simulink model "Function_Blocks"  (R2020b)
settings: Solver=FixedStepDiscrete  StartTime=0.0  StopTime=40  FixedStep=0.001  RelTol=1e-3
undefined symbols (not defined in the file): AA, C1, DiscIntNeverNeededParam, Error_Limit, kq, kqL
libraries: simulink x1, eeGeneralControl x1
(part 1 of 2)
settings Model: Creator=Jan Størbu  LastModifiedBy=Green Crane Testbed
settings DataIOCC: ReturnWorkspaceOutputs=off
settings DebuggingCC: BusObjectLabelMismatch=error  ArithmeticOperatorsInVariantConditions=warning
settings SFSimCC: SimUseLocalCustomCode=off  CustomCodeUndefinedFunction=UseInterfaceOnly
settings RTWCC: RTWUseLocalCustomCode=off
settings ConfigComp: PLC_TargetIDE=indraworks  PLC_ReuseMLFcnVariable=on  PLC_GenerateReport=off  PLC_LaunchReport=off

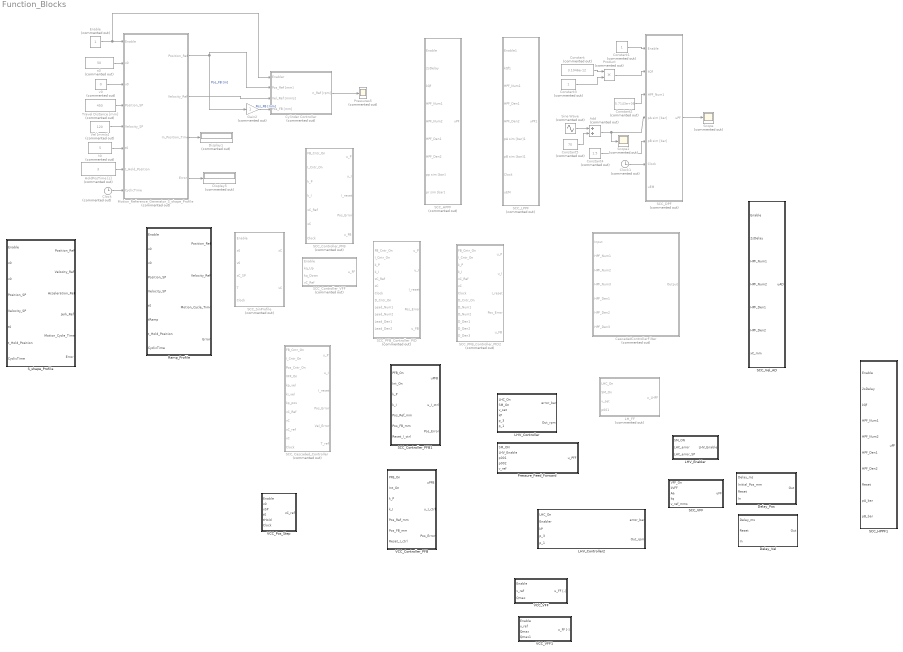
== system Function_Blocks ==
  Add : Sum  Commented=on
  CascadedControllerFilter : Subsystem  Commented=on  TreatAsAtomicUnit=on
  Clock : Clock  Commented=on
  Clock1 : Clock  Commented=on
  Constant : Constant  Commented=on  Value=3.1046e-12
  Constant1 : Constant  Commented=on  OutDataTypeStr=boolean
  Constant2 : Constant  Commented=on  Value=5.7143e+06
  Constant3 : Constant  Commented=on
  Constant4 : Constant  Commented=on  Value=1.5
  Constant5 : Constant  Commented=on  Value=70
  Cylinder Controller : Subsystem  Commented=on
  Delay_Pos : Subsystem  TreatAsAtomicUnit=on
  Delay_Vel : Subsystem  TreatAsAtomicUnit=on
  Display1 : Display  Commented=on
  Display5 : Display  Commented=on
  Enable : Constant  Commented=on  OutDataTypeStr=boolean
  Gain2 : Gain  Commented=on
  HoldPosTime [s] : Constant  Commented=on  Value=3
  "LHV_Controller " : Subsystem  TreatAsAtomicUnit=on
  LHV_Controller2 : Subsystem  TreatAsAtomicUnit=on
  LHV_Enabler : Subsystem  TreatAsAtomicUnit=on
  "LH_FF " : Subsystem  Commented=on
  Motion_Reference_Generator_S_shape_Profile : Subsystem  Commented=on  TreatAsAtomicUnit=on  VariantControl=S_shape_Profile
  Pressure_Feed_Forward : Subsystem  TreatAsAtomicUnit=on
  Pressures5 : Scope  Commented=on
  Product : Product  Commented=on
  Ramp_Profile : Subsystem  TreatAsAtomicUnit=on  VariantControl=Ramp_Profile
  SCC_Cascaded_Controller : Subsystem  Commented=on  TreatAsAtomicUnit=on
  SCC_Controller_PFB : Subsystem  Commented=on  TreatAsAtomicUnit=on
  SCC_Controller_PFB1 : Subsystem  TreatAsAtomicUnit=on
  SCC_Controller_VFF : Subsystem  Commented=on  TreatAsAtomicUnit=on
  SCC_DPF : Subsystem  Commented=on  TreatAsAtomicUnit=on
  SCC_HPPF : Subsystem  Commented=on  TreatAsAtomicUnit=on
  SCC_HPPF1 : Subsystem  TreatAsAtomicUnit=on
  SCC_LPPF : Subsystem  Commented=on  TreatAsAtomicUnit=on
  SCC_PFB_Controller_PID : Subsystem  Commented=on  TreatAsAtomicUnit=on
  SCC_PFB_Controller_PID2 : Subsystem  Commented=on  TreatAsAtomicUnit=on
  SCC_SinProfile : Subsystem  Commented=on  TreatAsAtomicUnit=on
  "SCC_VFF " : Subsystem  TreatAsAtomicUnit=on
  SCC_Vel_AD : Subsystem  TreatAsAtomicUnit=on
  S_shape_Profile : Subsystem  TreatAsAtomicUnit=on  VariantControl=S_shape_Profile
  Scope : Scope  Commented=on
  Scope1 : Scope  Commented=on
  Sine Wave : Sin  Commented=on  Amplitude=10  Frequency=14.5  SampleTime=0
  Travel Distance [mm] : Constant  Commented=on  Value=450
  VCC_Controller_PFB : Subsystem  TreatAsAtomicUnit=on
  VCC_Pos_Step : Subsystem  TreatAsAtomicUnit=on
  VCC_VFF : Subsystem  TreatAsAtomicUnit=on
  VCC_VFF1 : Subsystem  TreatAsAtomicUnit=on
  Vel [mm/s] : Constant  Commented=on  Value=120
  s0 : Constant  Commented=on  Value=50
  t0 : Constant  Commented=on  Value=5
  v0 : Constant  Commented=on  Value=0
  wires:
  Vel [mm/s]/1 -> Motion_Reference_Generator_S_shape_Profile/5(Velocity_SP)
  Gain2/1 -> Cylinder Controller/4(Pos_FB [mm])  "Pos_FB [mm]"
  Travel Distance [mm]/1 -> Motion_Reference_Generator_S_shape_Profile/4(Position_SP)
  Motion_Reference_Generator_S_shape_Profile/4(Error) -> Display5/1
  Enable/1 -> Motion_Reference_Generator_S_shape_Profile/1(Enable), Cylinder Controller/1(Enabler)
  Clock/1 -> Motion_Reference_Generator_S_shape_Profile/8(CyclicTime)
  Motion_Reference_Generator_S_shape_Profile/3(" In_Position_Time") -> Display1/1
  Motion_Reference_Generator_S_shape_Profile/2(Velocity_Ref) -> Cylinder Controller/3(Vel_Ref [mm/s])
  Motion_Reference_Generator_S_shape_Profile/1(Position_Ref) -> Cylinder Controller/2(Pos_Ref [mm]), Gain2/1  "Pos_FB [m]"
  s0/1 -> Motion_Reference_Generator_S_shape_Profile/2(x0)
  v0/1 -> Motion_Reference_Generator_S_shape_Profile/3(v0)
  HoldPosTime [s]/1 -> Motion_Reference_Generator_S_shape_Profile/7(t_Hold_Position)
  t0/1 -> Motion_Reference_Generator_S_shape_Profile/6(t0)
  Cylinder Controller/1(n_Ref [rpm]) -> Pressures5/1
  Constant/1 -> Product/1
  Sine Wave/1 -> Add/1
  SCC_DPF/1(uPF) -> Scope/1
  Constant4/1 -> SCC_DPF/5(pB sim [bar])
  Constant2/1 -> SCC_DPF/3(HPF_Num1)
  Add/1 -> Scope1/1, SCC_DPF/4(pA sim [bar])
  Constant5/1 -> Add/2
  Constant1/1 -> SCC_DPF/1(Enable)
  Clock1/1 -> SCC_DPF/6(Clock)
  Constant3/1 -> Product/2
  Product/1 -> SCC_DPF/2(kQf)

== system Function_Blocks/CascadedControllerFilter ==
  Input : Inport
  HPF_Num1 : Inport  Port=2
  HPF_Num2 : Inport  Port=3
  HPF_Num3 : Inport  Port=4
  HPF_Den1 : Inport  Port=5
  HPF_Den2 : Inport  Port=6
  HPF_Den3 : Inport  Port=7
  HP_Filter : DiscreteTransferFcn  NumeratorSource=Input port  Numerator=[3.786e-11 -3.786e-11]  DenominatorSource=Input port  Denominator=[1 -0.9954]  SampleTime=0.001  a0EqualsOne=on
      settings: InputPortMap=u0,p1,p3
  Vector Concatenate : Concatenate  NumInputs=3
  Vector Concatenate1 : Concatenate  NumInputs=3
  Output : Outport  VectorParamsAs1DForOutWhenUnconnected=off
  wires:
  HPF_Num1/1 -> Vector Concatenate/1
  Input/1 -> HP_Filter/1
  HPF_Num3/1 -> Vector Concatenate/3
  HPF_Den1/1 -> Vector Concatenate1/1
  HPF_Num2/1 -> Vector Concatenate/2
  HPF_Den3/1 -> Vector Concatenate1/3
  HPF_Den2/1 -> Vector Concatenate1/2
  Vector Concatenate1/1 -> HP_Filter/3
  Vector Concatenate/1 -> HP_Filter/2
  HP_Filter/1 -> Output/1

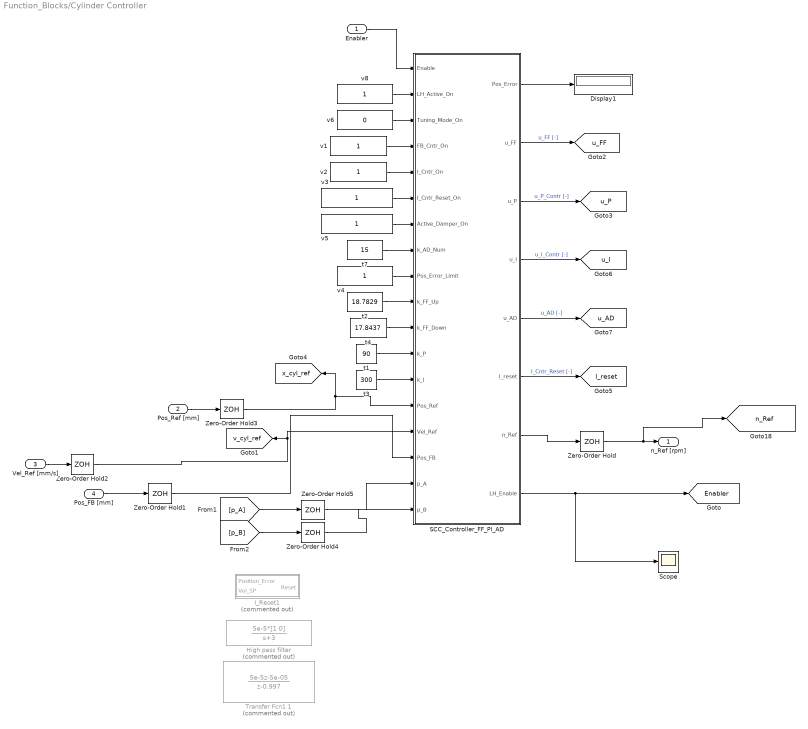
== system Function_Blocks/Cylinder Controller ==
  Enabler : Inport
  Pos_Ref [mm] : Inport  Port=2
  Vel_Ref [mm/s] : Inport  Port=3
  Pos_FB [mm] : Inport  Port=4
  Display1 : Display
  High pass filter : TransferFcn  Commented=on  Numerator=5e-5*[1 0]  Denominator=[1 3]
  I_Reset1 : Subsystem  Commented=on
  SCC_Controller_FF_PI_AD : Subsystem  TreatAsAtomicUnit=on
  Scope : Scope
  Transfer Fcn1 1 : DiscreteTransferFcn  Commented=on  Numerator=[5e-5 -5e-05]  Denominator=[1 -0.997]
  Zero-Order Hold{,1..5} (6 alike) : ZeroOrderHold  SampleTime=0.001
  t1 : Constant  Value=90
  t2 : Constant  Value=18.7829
  t3 : Constant  Value=300
  t4 : Constant  Value=17.8437
  t7 : Constant  Value=15
  v{1..3,5,8} (5 alike) : Constant  OutDataTypeStr=boolean
  v4 : Constant
  v6 : Constant  Value=0  OutDataTypeStr=boolean
  n_Ref [rpm] : Outport  VectorParamsAs1DForOutWhenUnconnected=off
  tag scope: Enabler=global, I_reset=global, n_Ref=global, u_AD=global, u_FF=global, u_I=global, u_P=global, v_cyl_ref=global, x_cyl_ref=global
  wires:
  v2/1 -> SCC_Controller_FF_PI_AD/5(I_Cntr_On)
  t3/1 -> SCC_Controller_FF_PI_AD/13(k_I)
  v1/1 -> SCC_Controller_FF_PI_AD/4(FB_Cntr_On)
  t1/1 -> SCC_Controller_FF_PI_AD/12(k_P)
  Pos_FB [mm]/1 -> Zero-Order Hold1/1
  SCC_Controller_FF_PI_AD/3(u_P) -> [u_P]  "u_P_Contr [-]"
  SCC_Controller_FF_PI_AD/2(u_FF) -> [u_FF]  "u_FF [-]"
  Pos_Ref [mm]/1 -> Zero-Order Hold3/1
  Vel_Ref [mm/s]/1 -> Zero-Order Hold2/1
  SCC_Controller_FF_PI_AD/6(I_reset) -> [I_reset]  "I_Cntr_Reset [-]"
  SCC_Controller_FF_PI_AD/1(Pos_Error) -> Display1/1
  SCC_Controller_FF_PI_AD/7(n_Ref) -> Zero-Order Hold/1
  SCC_Controller_FF_PI_AD/4(u_I) -> [u_I]  "u_I_Contr [-]"
  Zero-Order Hold/1 -> [n_Ref], n_Ref [rpm]/1
  Zero-Order Hold1/1 -> SCC_Controller_FF_PI_AD/16(Pos_FB)
  Zero-Order Hold2/1 -> SCC_Controller_FF_PI_AD/15(Vel_Ref), [v_cyl_ref]
  Zero-Order Hold3/1 -> SCC_Controller_FF_PI_AD/14(Pos_Ref), [x_cyl_ref]
  v3/1 -> SCC_Controller_FF_PI_AD/6(I_Cntr_Reset_On)
  v4/1 -> SCC_Controller_FF_PI_AD/9(Pos_Error_Limit)
  v5/1 -> SCC_Controller_FF_PI_AD/7(Active_Damper_On)
  [p_A] -> Zero-Order Hold5/1
  [p_B] -> Zero-Order Hold4/1
  Zero-Order Hold4/1 -> SCC_Controller_FF_PI_AD/18(p_B)
  Zero-Order Hold5/1 -> SCC_Controller_FF_PI_AD/17(p_A)
  SCC_Controller_FF_PI_AD/5(u_AD) -> [u_AD]  "u_AD [-]"
  t7/1 -> SCC_Controller_FF_PI_AD/8(k_AD_Num)
  v6/1 -> SCC_Controller_FF_PI_AD/3(Tuning_Mode_On)
  Enabler/1 -> SCC_Controller_FF_PI_AD/1(Enable)
  v8/1 -> SCC_Controller_FF_PI_AD/2(LH_Active_On)
  SCC_Controller_FF_PI_AD/8(LH_Enable) -> Scope/1, [Enabler]
  t2/1 -> SCC_Controller_FF_PI_AD/10(k_FF_Up)
  t4/1 -> SCC_Controller_FF_PI_AD/11(k_FF_Down)

== system Function_Blocks/Delay_Pos ==
  Delay_ms : Inport
  Initial_Pos_mm : Inport  Port=2
  Reset : Inport  Port=3  OutDataTypeStr=boolean
  In : Inport  Port=4
  Delay : Delay  DelayLengthSource=Input port  DelayLengthUpperLimit=200  InitialConditionSource=Input port  ExternalReset=Level hold  SampleTime=0.001
      settings: InputPortMap=u0,p1,r5,p4
  Out : Outport  VectorParamsAs1DForOutWhenUnconnected=off
  wires:
  Delay_ms/1 -> Delay/2
  Delay/1 -> Out/1
  In/1 -> Delay/1
  Reset/1 -> Delay/3
  Initial_Pos_mm/1 -> Delay/4

== system Function_Blocks/Delay_Vel ==
  Delay_ms : Inport
  Reset : Inport  Port=2  OutDataTypeStr=boolean
  In : Inport  Port=3
  Delay : Delay  DelayLengthSource=Input port  DelayLengthUpperLimit=200  ExternalReset=Level hold  SampleTime=0.001
      settings: InputPortMap=u0,p1,r5
  Out : Outport  VectorParamsAs1DForOutWhenUnconnected=off
  wires:
  Delay_ms/1 -> Delay/2
  Delay/1 -> Out/1
  In/1 -> Delay/1
  Reset/1 -> Delay/3

== system Function_Blocks/LHV_Controller  ==
  LHC_On : Inport  OutDataTypeStr=boolean
  SM_On : Inport  Port=2  OutDataTypeStr=boolean
  v_set : Inport  Port=3
  kP : Inport  Port=4
  p_3 : Inport  Port=5
  p_1 : Inport  Port=6
  1 : Gain  Gain=1e5
  12 : Gain  Gain=1e5
  Abs : Abs
  Add6 : Sum  Inputs=|+-
  Constant : Constant  Value=0
  Constant1 : Constant  Value=0
  Constant7 : Constant  Value=0
  Gain : Gain  Gain=1e-5
  Gain15 : Gain  Gain=60/(2*pi)
  Product : Product
  Saturation1 : Saturate  UpperLimit=1000  LowerLimit=-1000
  Switch1 : Switch  Criteria=u2 > Threshold
  Switch3 : Switch  Criteria=u2 > Threshold  OutDataTypeStr=boolean
  Switch5 : Switch  Criteria=u2 > Threshold
  Switch6 : Switch  Criteria=u2 > Threshold
  error_bar : Outport  VectorParamsAs1DForOutWhenUnconnected=off
  Out_rpm : Outport  Port=2  VectorParamsAs1DForOutWhenUnconnected=off
  wires:
  Product/1 -> Gain15/1  "Pa"
  Add6/1 -> Product/1, Gain/1  "FF+FB [rpm]"
  12/1 -> Add6/1
  Gain15/1 -> Switch1/1  "FF+FB [rpm]"
  p_3/1 -> Switch5/1  "[bar]"
  p_1/1 -> Switch6/1  "[bar]"
  1/1 -> Add6/2
  Constant/1 -> Switch1/3
  LHC_On/1 -> Switch1/2
  Switch1/1 -> Saturation1/1
  Saturation1/1 -> Out_rpm/1
  Constant7/1 -> Switch5/3, Switch6/3
  Switch3/1 -> Switch5/2, Switch6/2  "[bar]"
  Switch6/1 -> 1/1
  Switch5/1 -> 12/1
  Constant1/1 -> Switch3/1
  v_set/1 -> Abs/1
  Abs/1 -> Switch3/2
  SM_On/1 -> Switch3/3  "[bar]"
  Gain/1 -> error_bar/1
  kP/1 -> Product/2

== system Function_Blocks/LHV_Controller2 ==
  LHC_On : Inport  OutDataTypeStr=boolean
  Enabler : Inport  Port=2  OutDataTypeStr=boolean
  kP : Inport  Port=3
  p_3 : Inport  Port=4
  p_1 : Inport  Port=5
  1 : Gain  Gain=1e5
  12 : Gain  Gain=1e5
  Add1 : Sum  Inputs=|+-
  Add6 : Sum  Inputs=|+-
  Constant : Constant  Value=0
  Constant7 : Constant  Value=0
  Gain15 : Gain  Gain=60/(2*pi)
  Product : Product
  Saturation1 : Saturate  UpperLimit=1000  LowerLimit=0
  Switch1 : Switch  Criteria=u2 > Threshold
  Switch5 : Switch  Criteria=u2 > Threshold
  Switch6 : Switch  Criteria=u2 > Threshold
  "error_bar " : Outport  VectorParamsAs1DForOutWhenUnconnected=off
  Out_rpm : Outport  Port=2  VectorParamsAs1DForOutWhenUnconnected=off
  wires:
  Product/1 -> Gain15/1  "Pa"
  Add6/1 -> Product/1  "FF+FB [rpm]"
  12/1 -> Add6/1
  Gain15/1 -> Switch1/1  "FF+FB [rpm]"
  p_3/1 -> Add1/1, Switch5/1  "[bar]"
  p_1/1 -> Add1/2, Switch6/1  "[bar]"
  1/1 -> Add6/2
  Constant/1 -> Switch1/3
  LHC_On/1 -> Switch1/2
  Switch1/1 -> Saturation1/1
  Saturation1/1 -> Out_rpm/1
  Constant7/1 -> Switch5/3, Switch6/3
  Enabler/1 -> Switch5/2, Switch6/2  "[bar]"
  Switch6/1 -> 1/1
  Switch5/1 -> 12/1
  kP/1 -> Product/2
  Add1/1 -> "error_bar "/1  "FF+FB [rpm]"

== system Function_Blocks/LHV_Enabler ==
  SM_ON : Inport  OutDataTypeStr=boolean
  LHC_error : Inport  Port=2
  LHC_error_SP : Inport  Port=3
  MATLAB Function1 : MATLAB Function  TreatAsAtomicUnit=on
  LHV_Enable : Outport  VectorParamsAs1DForOutWhenUnconnected=off
  wires:
  MATLAB Function1/1(y) -> LHV_Enable/1
  SM_ON/1 -> MATLAB Function1/3(SM_ON)
  LHC_error/1 -> MATLAB Function1/1(LHC_error)
  LHC_error_SP/1 -> MATLAB Function1/2(LHC_error_SP)

== system Function_Blocks/LH_FF  ==
  LHC_On : Inport
  SM_On : Inport  Port=2
  v_set : Inport  Port=3
  p001 : Inport  Port=4
  12 : Gain  Gain=1e5
  Abs : Abs
  Constant : Constant  Value=0
  Constant7 : Constant  Value=0
  Switch1 : Switch  Criteria=u2 > Threshold
  Switch5 : Switch  Criteria=u2 > Threshold
  Transfer Fcn10 : TransferFcn  Numerator="[C1  kqL]"  Denominator=[0.002*kq kq ]
  u_LHFF : Outport  VectorParamsAs1DForOutWhenUnconnected=off
  wires:
  Transfer Fcn10/1 -> Switch1/1  "FF+FB [rpm]"
  p001/1 -> Switch5/1  "[bar]"
  Constant/1 -> Switch1/3
  LHC_On/1 -> Switch1/2
  Switch1/1 -> u_LHFF/1
  Constant7/1 -> Switch5/3
  Abs/1 -> Switch5/2  "[bar]"
  Switch5/1 -> 12/1
  12/1 -> Transfer Fcn10/1
  SM_On/1 -> ?  "[bar]"
  v_set/1 -> Abs/1  "[bar]"

== system Function_Blocks/Motion_Reference_Generator_S_shape_Profile ==
  Enable : Inport  OutDataTypeStr=boolean
  x0 : Inport  Port=2
  v0 : Inport  Port=3
  Position_SP : Inport  Port=4
  Velocity_SP : Inport  Port=5
  t0 : Inport  Port=6
  t_Hold_Position : Inport  Port=7
  CyclicTime : Inport  Port=8
  SP_Generator : MATLAB Function  TreatAsAtomicUnit=on
  Saturation : Saturate  UpperLimit=500  LowerLimit=0
  Saturation1 : Saturate  UpperLimit=150  LowerLimit=-150
  Saturation2 : Saturate  UpperLimit=150  LowerLimit=-150
  Saturation3 : Saturate  UpperLimit=500  LowerLimit=0
  Switch : Switch  Criteria=u2 > Threshold
  Switch1 : Switch  Criteria=u2 > Threshold
  Position_Ref : Outport  VectorParamsAs1DForOutWhenUnconnected=off
  Velocity_Ref : Outport  Port=2  VectorParamsAs1DForOutWhenUnconnected=off
  " In_Position_Time" : Outport  Port=3  VectorParamsAs1DForOutWhenUnconnected=off
  Error : Outport  Port=4  VectorParamsAs1DForOutWhenUnconnected=off
  wires:
  Saturation/1 -> SP_Generator/3(Desired_Position)
  Saturation1/1 -> SP_Generator/4(VelocitySP)
  t0/1 -> SP_Generator/5(t0)
  t_Hold_Position/1 -> SP_Generator/6(HoldPositionTime)
  Velocity_SP/1 -> Saturation1/1
  SP_Generator/3(InPositionTime) -> " In_Position_Time"/1
  CyclicTime/1 -> SP_Generator/7(t)
  SP_Generator/4(Error) -> Error/1
  Position_SP/1 -> Saturation/1
  Saturation2/1 -> Velocity_Ref/1
  Switch/1 -> Saturation2/1
  x0/1 -> Switch1/3, SP_Generator/1(s0)
  SP_Generator/1(PositionRef) -> Switch1/1
  Saturation3/1 -> Position_Ref/1
  v0/1 -> Switch/3, SP_Generator/2(v0)
  Enable/1 -> Switch1/2, Switch/2
  SP_Generator/2(VelocityRef) -> Switch/1
  Switch1/1 -> Saturation3/1

== system Function_Blocks/Pressure_Feed_Forward ==
  SM_ON : Inport  OutDataTypeStr=boolean
  LHV_Enable : Inport  Port=2  OutDataTypeStr=boolean
  p001 : Inport  Port=3
  p002 : Inport  Port=4
  v_ref : Inport  Port=5
  Constant : Constant  Value=0
  Gain2 : Gain  Gain=10^(5)
  Gain8 : Gain  Gain=10^(5)
  MATLAB Function1 : MATLAB Function  TreatAsAtomicUnit=on
  Subsystem2 : Subsystem
  Switch : Switch  Criteria=u2 > Threshold
  u_PFF : Outport  VectorParamsAs1DForOutWhenUnconnected=off
  wires:
  Subsystem2/1(p001_Hold) -> MATLAB Function1/1(p001_Hold)
  Gain8/1 -> MATLAB Function1/2(p_32)
  p002/1 -> Gain8/1
  v_ref/1 -> MATLAB Function1/3(x_dot_ref)
  p001/1 -> Gain2/1
  Switch/1 -> u_PFF/1
  LHV_Enable/1 -> Switch/2
  SM_ON/1 -> Subsystem2/Trigger
  Gain2/1 -> Subsystem2/1(p001)
  MATLAB Function1/1(FeedBackPressureTerm) -> Switch/1
  Constant/1 -> Switch/3

== system Function_Blocks/Ramp_Profile ==
  Enable : Inport  OutDataTypeStr=boolean
  x0 : Inport  Port=2
  v0 : Inport  Port=3
  Position_SP : Inport  Port=4
  Velocity_SP : Inport  Port=5
  t0 : Inport  Port=6
  tRamp : Inport  Port=7
  t_Hold_Position : Inport  Port=8
  CyclicTime : Inport  Port=9
  Saturation : Saturate  UpperLimit=150  LowerLimit=-150
  Saturation1 : Saturate  UpperLimit=500  LowerLimit=0
  Saturation2 : Saturate  UpperLimit=150  LowerLimit=0
  Saturation3 : Saturate  UpperLimit=500  LowerLimit=0
  Switch : Switch  Criteria=u2 > Threshold
  Switch1 : Switch  Criteria=u2 > Threshold
  WaveSignal : MATLAB Function  TreatAsAtomicUnit=on
  Position_Ref : Outport  VectorParamsAs1DForOutWhenUnconnected=off
  Velocity_Ref : Outport  Port=2  VectorParamsAs1DForOutWhenUnconnected=off
  Motion_Cycle_Time : Outport  Port=3  VectorParamsAs1DForOutWhenUnconnected=off
  Error : Outport  Port=4  VectorParamsAs1DForOutWhenUnconnected=off
  wires:
  CyclicTime/1 -> WaveSignal/8(t)
  WaveSignal/2(v) -> Switch/1
  Switch/1 -> Saturation/1
  v0/1 -> Switch/3, WaveSignal/2(v0)
  t0/1 -> WaveSignal/5(t0)
  Position_SP/1 -> Saturation3/1
  t_Hold_Position/1 -> WaveSignal/7(tWait)
  Velocity_SP/1 -> Saturation2/1
  WaveSignal/1(x) -> Switch1/1
  WaveSignal/3(T) -> Motion_Cycle_Time/1
  Enable/1 -> Switch1/2, Switch/2
  x0/1 -> Switch1/3, WaveSignal/1(x0)
  Switch1/1 -> Saturation1/1
  Saturation/1 -> Velocity_Ref/1
  Saturation1/1 -> Position_Ref/1
  WaveSignal/4(Error) -> Error/1
  Saturation2/1 -> WaveSignal/4(v_ref)
  Saturation3/1 -> WaveSignal/3(x_ref)
  tRamp/1 -> WaveSignal/6(tRamp)

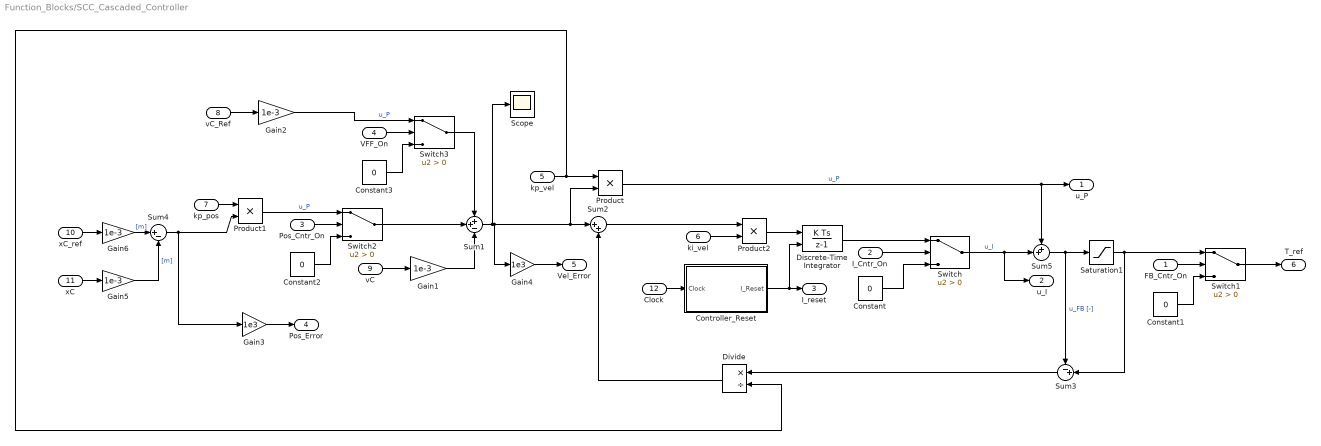
== system Function_Blocks/SCC_Cascaded_Controller ==
  FB_Cntr_On : Inport  OutDataTypeStr=boolean
  I_Cntr_On : Inport  Port=2  OutDataTypeStr=boolean
  Pos_Cntr_On : Inport  Port=3  OutDataTypeStr=boolean
  VFF_On : Inport  Port=4  OutDataTypeStr=boolean
  kp_vel : Inport  Port=5
  ki_vel : Inport  Port=6
  kp_pos : Inport  Port=7
  vC_Ref : Inport  Port=8
  vC : Inport  Port=9
  xC_ref : Inport  Port=10
  xC : Inport  Port=11
  Clock : Inport  Port=12
  Constant{,1..3} (4 alike) : Constant  Value=0
  Controller_Reset : MATLAB Function  TreatAsAtomicUnit=on
  Discrete-Time Integrator : DiscreteIntegrator  ExternalReset=sampled level  SampleTime=0.001  ICPrevOutput=DiscIntNeverNeededParam  ICPrevScaledInput=DiscIntNeverNeededParam
  Divide : Product  Inputs=*/
  Gain{1..2,5..6} (4 alike) : Gain  Gain=1e-3
  Gain3 : Gain  Gain=1e3
  Gain4 : Gain  Gain=1e3
  Product : Product
  Product1 : Product
  Product2 : Product
  Saturation1 : Saturate  UpperLimit=84  LowerLimit=-84
  Scope : Scope
  Sum1 : Sum  Inputs=++-
  Sum2 : Sum  Inputs=|++
  Sum3 : Sum  Inputs=-+|
  Sum4 : Sum  Inputs=|+-
  Sum5 : Sum  Inputs=++|
  Switch{,1..3} (4 alike) : Switch  Criteria=u2 > Threshold
  u_P : Outport  VectorParamsAs1DForOutWhenUnconnected=off
  u_I : Outport  Port=2  VectorParamsAs1DForOutWhenUnconnected=off
  I_reset : Outport  Port=3  VectorParamsAs1DForOutWhenUnconnected=off
  Pos_Error : Outport  Port=4  VectorParamsAs1DForOutWhenUnconnected=off
  Vel_Error : Outport  Port=5  VectorParamsAs1DForOutWhenUnconnected=off
  T_ref : Outport  Port=6  VectorParamsAs1DForOutWhenUnconnected=off
  wires:
  Product2/1 -> Discrete-Time Integrator/1
  vC/1 -> Gain1/1
  Product/1 -> Sum5/1, u_P/1  "u_P"
  Sum2/1 -> Product2/1
  Divide/1 -> Sum2/2
  kp_vel/1 -> Divide/2, Product/1
  ki_vel/1 -> Product2/2
  Discrete-Time Integrator/1 -> Switch/1
  Switch/1 -> Sum5/2, u_I/1  "u_I"
  I_Cntr_On/1 -> Switch/2
  Constant/1 -> Switch/3
  vC_Ref/1 -> Gain2/1
  Controller_Reset/1(I_Reset) -> I_reset/1, Discrete-Time Integrator/2
  Sum5/1 -> Saturation1/1, Sum3/1  "u_FB [-]"
  Sum3/1 -> Divide/1
  Constant1/1 -> Switch1/3
  FB_Cntr_On/1 -> Switch1/2
  Saturation1/1 -> Switch1/1, Sum3/2
  Clock/1 -> Controller_Reset/1(Clock)
  Switch1/1 -> T_ref/1
  Gain1/1 -> Sum1/3
  Pos_Cntr_On/1 -> Switch2/2
  Constant2/1 -> Switch2/3
  Product1/1 -> Switch2/1  "u_P"
  kp_pos/1 -> Product1/1
  xC/1 -> Gain5/1
  xC_ref/1 -> Gain6/1
  Gain3/1 -> Pos_Error/1
  Sum4/1 -> Gain3/1, Product1/2
  Sum1/1 -> Scope/1, Gain4/1, Product/2, Sum2/1
  Gain4/1 -> Vel_Error/1
  Gain5/1 -> Sum4/2  "[m]"
  Gain6/1 -> Sum4/1  "[m]"
  Switch2/1 -> Sum1/2
  VFF_On/1 -> Switch3/2
  Constant3/1 -> Switch3/3
  Gain2/1 -> Switch3/1  "u_P"
  Switch3/1 -> Sum1/1

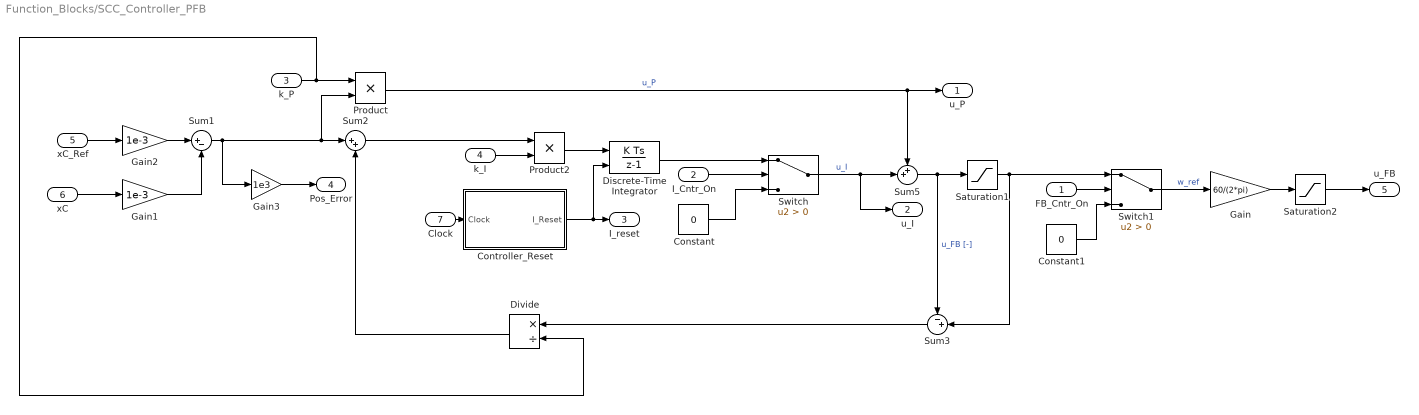
== system Function_Blocks/SCC_Controller_PFB ==
  FB_Cntr_On : Inport  OutDataTypeStr=boolean
  I_Cntr_On : Inport  Port=2  OutDataTypeStr=boolean
  k_P : Inport  Port=3
  k_I : Inport  Port=4
  xC_Ref : Inport  Port=5
  xC : Inport  Port=6
  Clock : Inport  Port=7
  Constant : Constant  Value=0
  Constant1 : Constant  Value=0
  Controller_Reset : MATLAB Function  TreatAsAtomicUnit=on
  Discrete-Time Integrator : DiscreteIntegrator  ExternalReset=sampled level  SampleTime=0.001  ICPrevOutput=DiscIntNeverNeededParam  ICPrevScaledInput=DiscIntNeverNeededParam
  Divide : Product  Inputs=*/
  Gain : Gain  Gain=60/(2*pi)
  Gain1 : Gain  Gain=1e-3
  Gain2 : Gain  Gain=1e-3
  Gain3 : Gain  Gain=1e3
  Product : Product
  Product2 : Product
  Saturation1 : Saturate  UpperLimit=3600*(2*pi)/60  LowerLimit=-3600*(2*pi)/60
  Saturation2 : Saturate  UpperLimit=3600  LowerLimit=-3600
  Sum1 : Sum  Inputs=|+-
  Sum2 : Sum  Inputs=|++
  Sum3 : Sum  Inputs=-+|
  Sum5 : Sum  Inputs=++|
  Switch : Switch  Criteria=u2 > Threshold
  Switch1 : Switch  Criteria=u2 > Threshold
  u_P : Outport  VectorParamsAs1DForOutWhenUnconnected=off
  u_I : Outport  Port=2  VectorParamsAs1DForOutWhenUnconnected=off
  I_reset : Outport  Port=3  VectorParamsAs1DForOutWhenUnconnected=off
  Pos_Error : Outport  Port=4  VectorParamsAs1DForOutWhenUnconnected=off
  u_FB : Outport  Port=5  VectorParamsAs1DForOutWhenUnconnected=off
  wires:
  Product2/1 -> Discrete-Time Integrator/1
  xC/1 -> Gain1/1
  Product/1 -> Sum5/1, u_P/1  "u_P"
  Sum2/1 -> Product2/1
  Divide/1 -> Sum2/2
  k_P/1 -> Divide/2, Product/1
  k_I/1 -> Product2/2
  Sum1/1 -> Product/2, Sum2/1, Gain3/1
  Discrete-Time Integrator/1 -> Switch/1
  Switch/1 -> Sum5/2, u_I/1  "u_I"
  I_Cntr_On/1 -> Switch/2
  Constant/1 -> Switch/3
  xC_Ref/1 -> Gain2/1
  Controller_Reset/1(I_Reset) -> I_reset/1, Discrete-Time Integrator/2
  Sum5/1 -> Saturation1/1, Sum3/1  "u_FB [-]"
  Sum3/1 -> Divide/1
  Switch1/1 -> Gain/1  "w_ref"
  Constant1/1 -> Switch1/3
  FB_Cntr_On/1 -> Switch1/2
  Saturation1/1 -> Switch1/1, Sum3/2
  Clock/1 -> Controller_Reset/1(Clock)
  Saturation2/1 -> u_FB/1
  Gain/1 -> Saturation2/1
  Gain1/1 -> Sum1/2
  Gain2/1 -> Sum1/1
  Gain3/1 -> Pos_Error/1

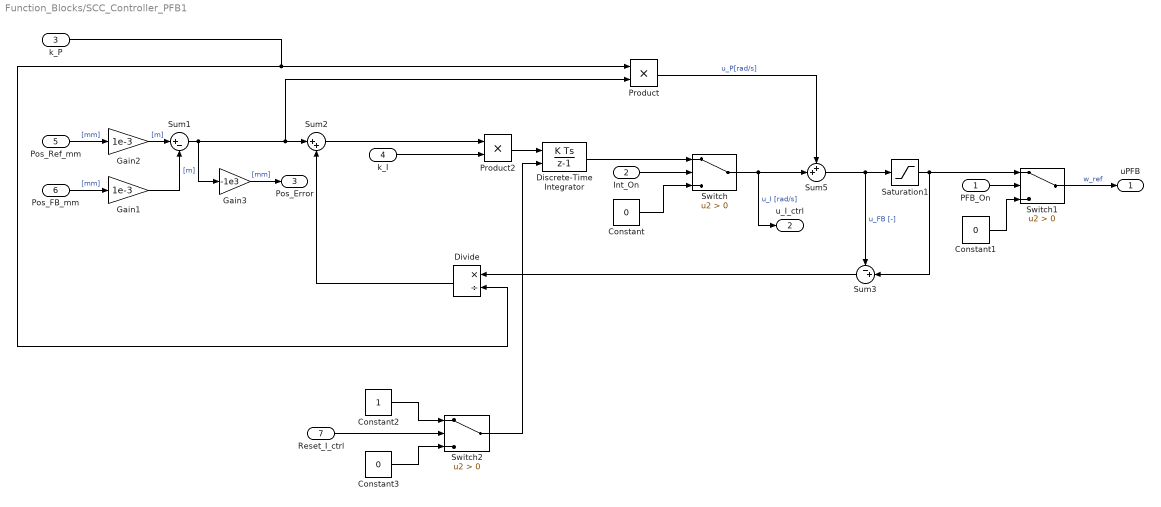
== system Function_Blocks/SCC_Controller_PFB1 ==
  PFB_On : Inport  OutDataTypeStr=boolean
  Int_On : Inport  Port=2  OutDataTypeStr=boolean
  k_P : Inport  Port=3
  k_I : Inport  Port=4
  Pos_Ref_mm : Inport  Port=5
  Pos_FB_mm : Inport  Port=6
  Reset_I_ctrl : Inport  Port=7  OutDataTypeStr=boolean
  Constant : Constant  Value=0
  Constant1 : Constant  Value=0
  Constant2 : Constant
  Constant3 : Constant  Value=0
  Discrete-Time Integrator : DiscreteIntegrator  ExternalReset=sampled level  SampleTime=0.001  ICPrevOutput=DiscIntNeverNeededParam  ICPrevScaledInput=DiscIntNeverNeededParam
  Divide : Product  Inputs=*/
  Gain1 : Gain  Gain=1e-3
  Gain2 : Gain  Gain=1e-3
  Gain3 : Gain  Gain=-1e3
  Product : Product
  Product2 : Product
  Saturation1 : Saturate  UpperLimit=3200  LowerLimit=-3200
  Sum1 : Sum  Inputs=|+-
  Sum2 : Sum  Inputs=|++
  Sum3 : Sum  Inputs=-+|
  Sum5 : Sum  Inputs=++|
  Switch : Switch  Criteria=u2 > Threshold
  Switch1 : Switch  Criteria=u2 > Threshold
  Switch2 : Switch  Criteria=u2 > Threshold
  uPFB : Outport  VectorParamsAs1DForOutWhenUnconnected=off
  u_I_ctrl : Outport  Port=2  VectorParamsAs1DForOutWhenUnconnected=off
  Pos_Error : Outport  Port=3  VectorParamsAs1DForOutWhenUnconnected=off
  wires:
  Pos_FB_mm/1 -> Gain1/1  "[mm]"
  Sum2/1 -> Product2/1
  Divide/1 -> Sum2/2
  k_P/1 -> Product/1, Divide/2
  k_I/1 -> Product2/2
  Sum1/1 -> Product/2, Sum2/1, Gain3/1
  Int_On/1 -> Switch/2
  Constant/1 -> Switch/3
  Pos_Ref_mm/1 -> Gain2/1  "[mm]"
  Sum5/1 -> Sum3/1, Saturation1/1  "u_FB [-]"
  Sum3/1 -> Divide/1
  Switch1/1 -> uPFB/1  "w_ref"
  Constant1/1 -> Switch1/3
  PFB_On/1 -> Switch1/2
  Saturation1/1 -> Switch1/1, Sum3/2
  Gain1/1 -> Sum1/2  "[m]"
  Gain2/1 -> Sum1/1  "[m]"
  Gain3/1 -> Pos_Error/1  "[mm]"
  Product/1 -> Sum5/1  "u_P[rad/s]"
  Switch/1 -> u_I_ctrl/1, Sum5/2  "u_I [rad/s]"
  Product2/1 -> Discrete-Time Integrator/1
  Reset_I_ctrl/1 -> Switch2/2
  Switch2/1 -> Discrete-Time Integrator/2
  Discrete-Time Integrator/1 -> Switch/1
  Constant2/1 -> Switch2/1
  Constant3/1 -> Switch2/3

== system Function_Blocks/SCC_Controller_VFF ==
  Enable : Inport  OutDataTypeStr=boolean
  kq_Up : Inport  Port=2
  kq_Down : Inport  Port=3
  vC_Ref : Inport  Port=4
  Constant : Constant  Value=0
  Divide1 : Product  Inputs=*/
  Divide2 : Product  Inputs=*/
  Gain1 : Gain  Gain=1e-3
  Gain3 : Gain  Gain=AA
  Switch : Switch
  Switch1 : Switch  Criteria=u2 > Threshold
  u_FF : Outport  VectorParamsAs1DForOutWhenUnconnected=off
  wires:
  Divide2/1 -> Switch/3  "[rev/min]"
  Divide1/1 -> Switch/1  "[rev/min]"
  vC_Ref/1 -> Gain1/1
  kq_Up/1 -> Divide1/2
  kq_Down/1 -> Divide2/2
  Gain1/1 -> Gain3/1
  Gain3/1 -> Divide2/1, Divide1/1, Switch/2
  Switch/1 -> Switch1/1
  Switch1/1 -> u_FF/1
  Enable/1 -> Switch1/2
  Constant/1 -> Switch1/3

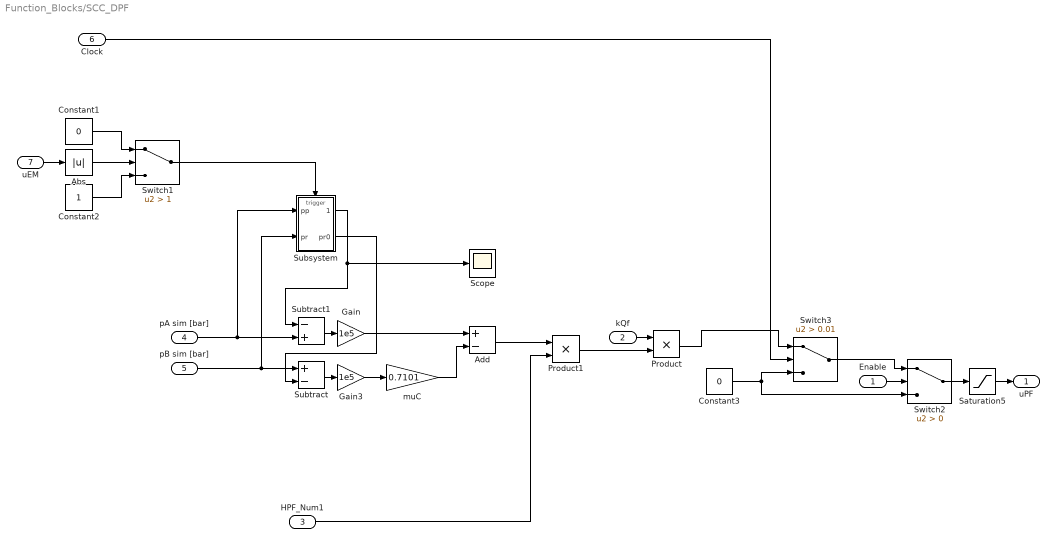
== system Function_Blocks/SCC_DPF ==
  Enable : Inport  OutDataTypeStr=boolean
  kQf : Inport  Port=2
  HPF_Num1 : Inport  Port=3
  pA sim [bar] : Inport  Port=4
  pB sim [bar] : Inport  Port=5
  Clock : Inport  Port=6
  uEM : Inport  Port=7
  Abs : Abs
  Add : Sum  Inputs=+-
  Constant1 : Constant  Value=0
  Constant2 : Constant
  Constant3 : Constant  Value=0
  Gain : Gain  Gain=1e5
  Gain3 : Gain  Gain=1e5
  Product : Product
  Product1 : Product
  Saturation5 : Saturate  UpperLimit=3600  LowerLimit=-3600
  Scope : Scope
  Subsystem : Subsystem
  Subtract : Sum  Inputs=+-
  Subtract1 : Sum  Inputs=-+
  Switch1 : Switch  Criteria=u2 > Threshold  Threshold=1
  Switch2 : Switch  Criteria=u2 > Threshold
  Switch3 : Switch  Criteria=u2 > Threshold  Threshold=0.01
  muC : Gain  Gain=0.7101
  uPF : Outport  VectorParamsAs1DForOutWhenUnconnected=off
  wires:
  Add/1 -> Product1/1
  Gain/1 -> Add/1
  Product1/1 -> Product/2
  Constant3/1 -> Switch2/3, Switch3/3
  Gain3/1 -> muC/1
  HPF_Num1/1 -> Product1/2
  Switch2/1 -> Saturation5/1
  Enable/1 -> Switch2/2
  Saturation5/1 -> uPF/1
  kQf/1 -> Product/1
  muC/1 -> Add/2
  Subtract/1 -> Gain3/1
  pB sim [bar]/1 -> Subsystem/2(pr), Subtract/1
  Subsystem/2(pr0) -> Subtract/2
  Subtract1/1 -> Gain/1
  pA sim [bar]/1 -> Subsystem/1(pp), Subtract1/2
  Subsystem/1(pp0) -> Subtract1/1, Scope/1
  Clock/1 -> Switch3/2
  Constant1/1 -> Switch1/1
  Constant2/1 -> Switch1/3
  Switch1/1 -> Subsystem/Trigger
  Product/1 -> Switch3/1
  Switch3/1 -> Switch2/1
  uEM/1 -> Abs/1
  Abs/1 -> Switch1/2

== system Function_Blocks/SCC_HPPF ==
  Enable : Inport  OutDataTypeStr=boolean
  2sDelay : Inport  Port=2
  kQf : Inport  Port=3
  HPF_Num1 : Inport  Port=4
  HPF_Num2 : Inport  Port=5
  HPF_Den1 : Inport  Port=6
  HPF_Den2 : Inport  Port=7
  pp sim [bar] : Inport  Port=8
  pr sim [bar] : Inport  Port=9
  Add : Sum  Inputs=+-
  Constant : Constant  Value=0
  Gain : Gain  Gain=1e5
  Gain3 : Gain  Gain=1e5
  HP_Filter : DiscreteTransferFcn  NumeratorSource=Input port  Numerator=[3.786e-11 -3.786e-11]  DenominatorSource=Input port  Denominator=[1 -0.9954]  SampleTime=0.001  a0EqualsOne=on
      settings: InputPortMap=u0,p1,p3
  Product : Product
  Saturation5 : Saturate  UpperLimit=3600  LowerLimit=-3600
  Switch1 : Switch  Criteria=u2 > Threshold  Threshold=2
  Switch2 : Switch  Criteria=u2 > Threshold
  Vector Concatenate : Concatenate
  Vector Concatenate1 : Concatenate
  muC : Gain  Gain=0.7101
  uPF : Outport  VectorParamsAs1DForOutWhenUnconnected=off
  wires:
  pr sim [bar]/1 -> Gain3/1
  pp sim [bar]/1 -> Gain/1
  Add/1 -> HP_Filter/1
  Gain/1 -> Add/1
  HP_Filter/1 -> Product/2
  Constant/1 -> Switch2/3, Switch1/3
  Gain3/1 -> muC/1
  Vector Concatenate/1 -> HP_Filter/2
  Vector Concatenate1/1 -> HP_Filter/3
  HPF_Num1/1 -> Vector Concatenate/1
  HPF_Num2/1 -> Vector Concatenate/2
  HPF_Den1/1 -> Vector Concatenate1/1
  HPF_Den2/1 -> Vector Concatenate1/2
  Switch2/1 -> Saturation5/1
  Switch1/1 -> Switch2/1
  Enable/1 -> Switch2/2
  Saturation5/1 -> uPF/1
  2sDelay/1 -> Switch1/2
  Product/1 -> Switch1/1
  kQf/1 -> Product/1
  muC/1 -> Add/2

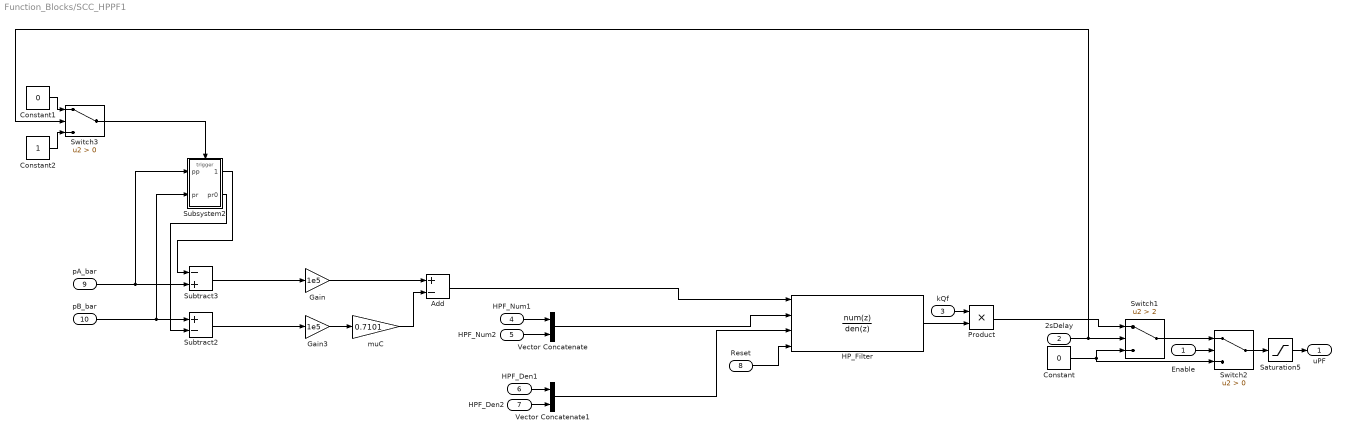
== system Function_Blocks/SCC_HPPF1 ==
  Enable : Inport  OutDataTypeStr=boolean
  2sDelay : Inport  Port=2
  kQf : Inport  Port=3
  HPF_Num1 : Inport  Port=4
  HPF_Num2 : Inport  Port=5
  HPF_Den1 : Inport  Port=6
  HPF_Den2 : Inport  Port=7
  Reset : Inport  Port=8  OutDataTypeStr=boolean
  pA_bar : Inport  Port=9
  pB_bar : Inport  Port=10
  Add : Sum  Inputs=+-
  Constant : Constant  Value=0
  Constant1 : Constant  Value=0
  Constant2 : Constant
  Gain : Gain  Gain=1e5
  Gain3 : Gain  Gain=1e5
  HP_Filter : DiscreteTransferFcn  NumeratorSource=Input port  Numerator=[3.786e-11 -3.786e-11]  DenominatorSource=Input port  Denominator=[1 -0.9954]  ExternalReset=Level hold  SampleTime=0.001  a0EqualsOne=on
      settings: InputPortMap=u0,p1,p3,r7
  Product : Product
  Saturation5 : Saturate  UpperLimit=3600  LowerLimit=-3600
  Subsystem2 : Subsystem
  Subtract2 : Sum  Inputs=+-
  Subtract3 : Sum  Inputs=-+
  Switch1 : Switch  Criteria=u2 > Threshold  Threshold=2
  Switch2 : Switch  Criteria=u2 > Threshold
  Switch3 : Switch  Criteria=u2 > Threshold
  Vector Concatenate : Concatenate
  Vector Concatenate1 : Concatenate
  muC : Gain  Gain=0.7101
  uPF : Outport  VectorParamsAs1DForOutWhenUnconnected=off
  wires:
  Add/1 -> HP_Filter/1
  Gain/1 -> Add/1
  HP_Filter/1 -> Product/2
  Constant/1 -> Switch2/3, Switch1/3
  Gain3/1 -> muC/1
  Vector Concatenate/1 -> HP_Filter/2
  Vector Concatenate1/1 -> HP_Filter/3
  HPF_Num1/1 -> Vector Concatenate/1
  HPF_Num2/1 -> Vector Concatenate/2
  HPF_Den1/1 -> Vector Concatenate1/1
  HPF_Den2/1 -> Vector Concatenate1/2
  Switch2/1 -> Saturation5/1
  Switch1/1 -> Switch2/1
  Enable/1 -> Switch2/2
  Saturation5/1 -> uPF/1
  Product/1 -> Switch1/1
  kQf/1 -> Product/1
  muC/1 -> Add/2
  pA_bar/1 -> Subsystem2/1(pp), Subtract3/2
  Subtract2/1 -> Gain3/1
  pB_bar/1 -> Subsystem2/2(pr), Subtract2/1
  Subtract3/1 -> Gain/1
  Subsystem2/2(pr0) -> Subtract2/2
  Subsystem2/1(pp0) -> Subtract3/1
  Constant1/1 -> Switch3/1
  2sDelay/1 -> Switch3/2, Switch1/2
  Constant2/1 -> Switch3/3
  Switch3/1 -> Subsystem2/Trigger
  Reset/1 -> HP_Filter/4

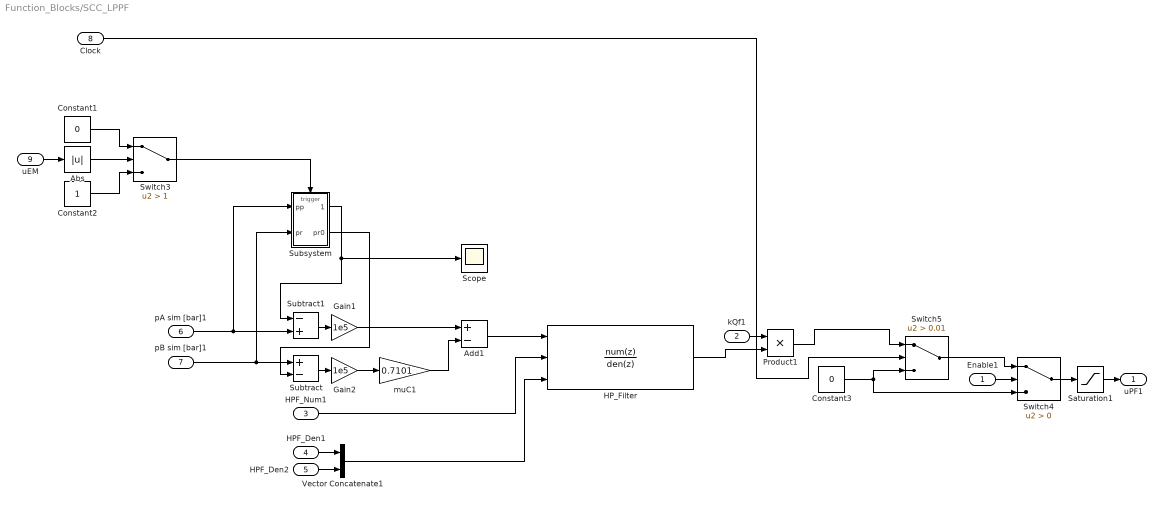
== system Function_Blocks/SCC_LPPF ==
  Enable1 : Inport  OutDataTypeStr=boolean
  kQf1 : Inport  Port=2
  HPF_Num1 : Inport  Port=3
  HPF_Den1 : Inport  Port=4
  HPF_Den2 : Inport  Port=5
  pA sim [bar]1 : Inport  Port=6
  pB sim [bar]1 : Inport  Port=7
  Clock : Inport  Port=8
  uEM : Inport  Port=9
  Abs : Abs
  Add1 : Sum  Inputs=+-
  Constant1 : Constant  Value=0
  Constant2 : Constant
  Constant3 : Constant  Value=0
  Gain1 : Gain  Gain=1e5
  Gain2 : Gain  Gain=1e5
  HP_Filter : DiscreteTransferFcn  NumeratorSource=Input port  Numerator=[3.786e-11]  DenominatorSource=Input port  Denominator=[1 -0.9954]  SampleTime=0.001  a0EqualsOne=on
      settings: InputPortMap=u0,p1,p3
  Product1 : Product
  Saturation1 : Saturate  UpperLimit=3600  LowerLimit=-3600
  Scope : Scope
  Subsystem : Subsystem
  Subtract : Sum  Inputs=+-
  Subtract1 : Sum  Inputs=-+
  Switch3 : Switch  Criteria=u2 > Threshold  Threshold=1
  Switch4 : Switch  Criteria=u2 > Threshold
  Switch5 : Switch  Criteria=u2 > Threshold  Threshold=0.01
  Vector Concatenate1 : Concatenate
  muC1 : Gain  Gain=0.7101
  uPF1 : Outport  VectorParamsAs1DForOutWhenUnconnected=off
  wires:
  Add1/1 -> HP_Filter/1
  HPF_Num1/1 -> HP_Filter/2
  Vector Concatenate1/1 -> HP_Filter/3
  HPF_Den1/1 -> Vector Concatenate1/1
  HPF_Den2/1 -> Vector Concatenate1/2
  uEM/1 -> Abs/1
  Constant3/1 -> Switch4/3, Switch5/3
  Switch5/1 -> Switch4/1
  Product1/1 -> Switch5/1
  Abs/1 -> Switch3/2
  Subsystem/1(pp0) -> Subtract1/1, Scope/1
  Subtract1/1 -> Gain1/1
  HP_Filter/1 -> Product1/2
  Subtract/1 -> Gain2/1
  pA sim [bar]1/1 -> Subsystem/1(pp), Subtract1/2
  Switch3/1 -> Subsystem/Trigger
  Constant2/1 -> Switch3/3
  Constant1/1 -> Switch3/1
  Clock/1 -> Switch5/2
  Subsystem/2(pr0) -> Subtract/2
  Saturation1/1 -> uPF1/1
  Gain1/1 -> Add1/1
  Enable1/1 -> Switch4/2
  kQf1/1 -> Product1/1
  pB sim [bar]1/1 -> Subsystem/2(pr), Subtract/1
  Gain2/1 -> muC1/1
  muC1/1 -> Add1/2
  Switch4/1 -> Saturation1/1

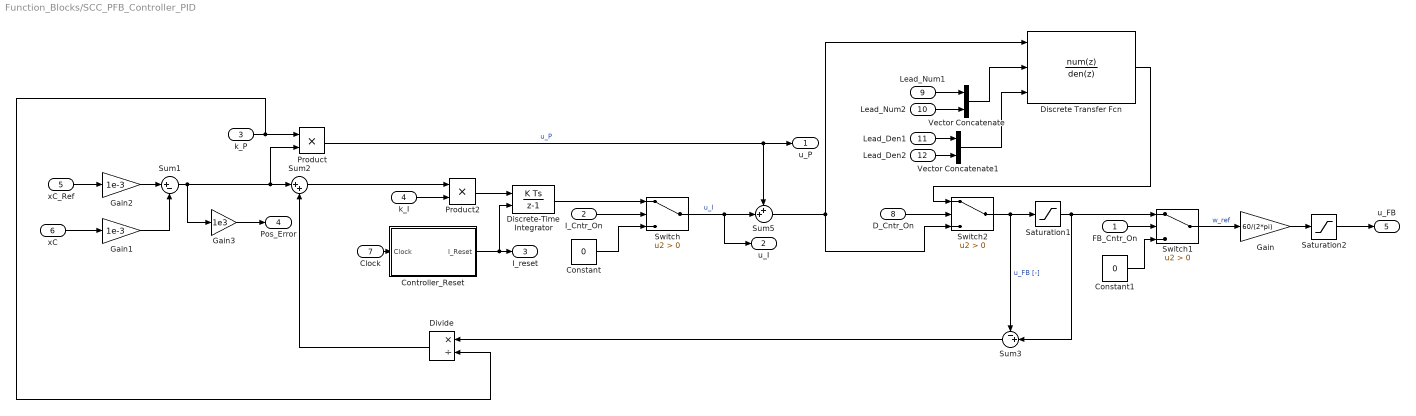
== system Function_Blocks/SCC_PFB_Controller_PID ==
  FB_Cntr_On : Inport  OutDataTypeStr=boolean
  I_Cntr_On : Inport  Port=2  OutDataTypeStr=boolean
  k_P : Inport  Port=3
  k_I : Inport  Port=4
  xC_Ref : Inport  Port=5
  xC : Inport  Port=6
  Clock : Inport  Port=7
  D_Cntr_On : Inport  Port=8  OutDataTypeStr=boolean
  Lead_Num1 : Inport  Port=9
  Lead_Num2 : Inport  Port=10
  Lead_Den1 : Inport  Port=11
  Lead_Den2 : Inport  Port=12
  Constant : Constant  Value=0
  Constant1 : Constant  Value=0
  Controller_Reset : MATLAB Function  TreatAsAtomicUnit=on
  Discrete Transfer Fcn : DiscreteTransferFcn  NumeratorSource=Input port  Numerator=[1 1]  DenominatorSource=Input port  Denominator=[1 1]  a0EqualsOne=on
      settings: InputPortMap=u0,p1,p3
  Discrete-Time Integrator : DiscreteIntegrator  ExternalReset=sampled level  SampleTime=0.001  ICPrevOutput=DiscIntNeverNeededParam  ICPrevScaledInput=DiscIntNeverNeededParam
  Divide : Product  Inputs=*/
  Gain : Gain  Gain=60/(2*pi)
  Gain1 : Gain  Gain=1e-3
  Gain2 : Gain  Gain=1e-3
  Gain3 : Gain  Gain=1e3
  Product : Product
  Product2 : Product
  Saturation1 : Saturate  UpperLimit=3600*(2*pi)/60  LowerLimit=-3600*(2*pi)/60
  Saturation2 : Saturate  UpperLimit=3600  LowerLimit=-3600
  Sum1 : Sum  Inputs=|+-
  Sum2 : Sum  Inputs=|++
  Sum3 : Sum  Inputs=-+|
  Sum5 : Sum  Inputs=++|
  Switch : Switch  Criteria=u2 > Threshold
  Switch1 : Switch  Criteria=u2 > Threshold
  Switch2 : Switch  Criteria=u2 > Threshold
  Vector Concatenate : Concatenate
  Vector Concatenate1 : Concatenate
  u_P : Outport  VectorParamsAs1DForOutWhenUnconnected=off
  u_I : Outport  Port=2  VectorParamsAs1DForOutWhenUnconnected=off
  I_reset : Outport  Port=3  VectorParamsAs1DForOutWhenUnconnected=off
  Pos_Error : Outport  Port=4  VectorParamsAs1DForOutWhenUnconnected=off
  u_FB : Outport  Port=5  VectorParamsAs1DForOutWhenUnconnected=off
  wires:
  Product2/1 -> Discrete-Time Integrator/1
  xC/1 -> Gain1/1
  Product/1 -> Sum5/1, u_P/1  "u_P"
  Sum2/1 -> Product2/1
  Divide/1 -> Sum2/2
  k_P/1 -> Divide/2, Product/1
  k_I/1 -> Product2/2
  Sum1/1 -> Product/2, Sum2/1, Gain3/1
  Discrete-Time Integrator/1 -> Switch/1
  Switch/1 -> Sum5/2, u_I/1  "u_I"
  I_Cntr_On/1 -> Switch/2
  Constant/1 -> Switch/3
  xC_Ref/1 -> Gain2/1
  Controller_Reset/1(I_Reset) -> I_reset/1, Discrete-Time Integrator/2
  Sum3/1 -> Divide/1
  Clock/1 -> Controller_Reset/1(Clock)
  Gain1/1 -> Sum1/2
  Gain2/1 -> Sum1/1
  Gain3/1 -> Pos_Error/1
  Lead_Den2/1 -> Vector Concatenate1/2
  Lead_Num2/1 -> Vector Concatenate/2
  Vector Concatenate/1 -> Discrete Transfer Fcn/2
  Lead_Num1/1 -> Vector Concatenate/1
  Vector Concatenate1/1 -> Discrete Transfer Fcn/3
  Lead_Den1/1 -> Vector Concatenate1/1
  D_Cntr_On/1 -> Switch2/2
  Discrete Transfer Fcn/1 -> Switch2/1
  Sum5/1 -> Discrete Transfer Fcn/1, Switch2/3
  Saturation2/1 -> u_FB/1
  Constant1/1 -> Switch1/3
  Saturation1/1 -> Switch1/1, Sum3/2
  Gain/1 -> Saturation2/1
  FB_Cntr_On/1 -> Switch1/2
  Switch1/1 -> Gain/1  "w_ref"
  Switch2/1 -> Saturation1/1, Sum3/1  "u_FB [-]"

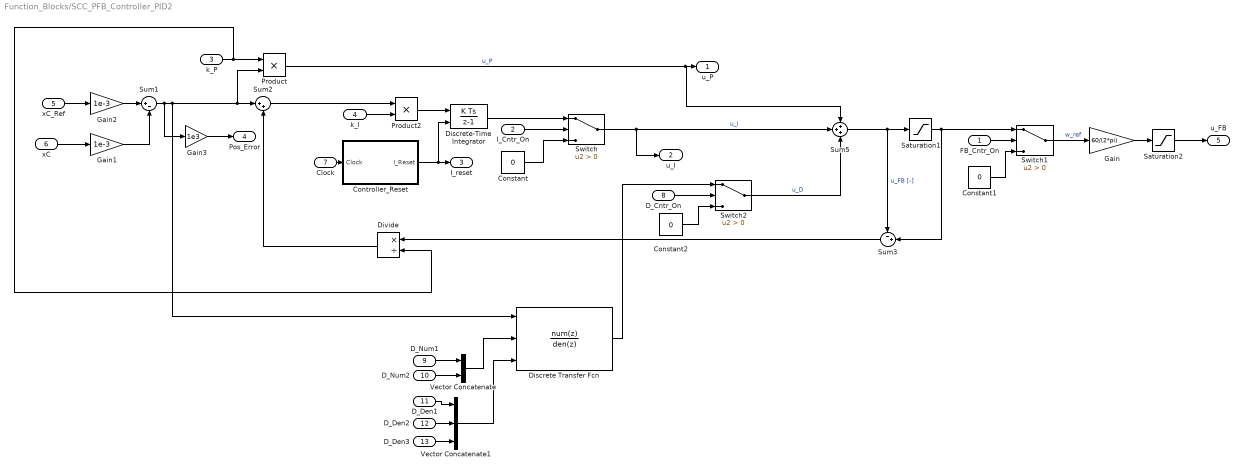
== system Function_Blocks/SCC_PFB_Controller_PID2 ==
  FB_Cntr_On : Inport  OutDataTypeStr=boolean
  I_Cntr_On : Inport  Port=2  OutDataTypeStr=boolean
  k_P : Inport  Port=3
  k_I : Inport  Port=4
  xC_Ref : Inport  Port=5
  xC : Inport  Port=6
  Clock : Inport  Port=7
  D_Cntr_On : Inport  Port=8  OutDataTypeStr=boolean
  D_Num1 : Inport  Port=9
  D_Num2 : Inport  Port=10
  D_Den1 : Inport  Port=11
  D_Den2 : Inport  Port=12
  D_Den3 : Inport  Port=13
  Constant : Constant  Value=0
  Constant1 : Constant  Value=0
  Constant2 : Constant  Value=0
  Controller_Reset : MATLAB Function  TreatAsAtomicUnit=on
  Discrete Transfer Fcn : DiscreteTransferFcn  NumeratorSource=Input port  Numerator=[1 1]  DenominatorSource=Input port  Denominator=[1 1]  a0EqualsOne=on
      settings: InputPortMap=u0,p1,p3
  Discrete-Time Integrator : DiscreteIntegrator  ExternalReset=sampled level  SampleTime=0.001  ICPrevOutput=DiscIntNeverNeededParam  ICPrevScaledInput=DiscIntNeverNeededParam
  Divide : Product  Inputs=*/
  Gain : Gain  Gain=60/(2*pi)
  Gain1 : Gain  Gain=1e-3
  Gain2 : Gain  Gain=1e-3
  Gain3 : Gain  Gain=1e3
  Product : Product
  Product2 : Product
  Saturation1 : Saturate  UpperLimit=3200*(2*pi)/60  LowerLimit=-3200*(2*pi)/60
  Saturation2 : Saturate  UpperLimit=3200  LowerLimit=-3200
  Sum1 : Sum  Inputs=|+-
  Sum2 : Sum  Inputs=|++
  Sum3 : Sum  Inputs=-+|
  Sum5 : Sum  Inputs=+++
  Switch : Switch  Criteria=u2 > Threshold
  Switch1 : Switch  Criteria=u2 > Threshold
  Switch2 : Switch  Criteria=u2 > Threshold
  Vector Concatenate : Concatenate
  Vector Concatenate1 : Concatenate  NumInputs=3
  u_P : Outport  VectorParamsAs1DForOutWhenUnconnected=off
  u_I : Outport  Port=2  VectorParamsAs1DForOutWhenUnconnected=off
  I_reset : Outport  Port=3  VectorParamsAs1DForOutWhenUnconnected=off
  Pos_Error : Outport  Port=4  VectorParamsAs1DForOutWhenUnconnected=off
  u_FB : Outport  Port=5  VectorParamsAs1DForOutWhenUnconnected=off
  wires:
  Product2/1 -> Discrete-Time Integrator/1
  xC/1 -> Gain1/1
  Product/1 -> Sum5/1, u_P/1  "u_P"
  Sum2/1 -> Product2/1
  Divide/1 -> Sum2/2
  k_P/1 -> Divide/2, Product/1
  k_I/1 -> Product2/2
  Discrete-Time Integrator/1 -> Switch/1
  Switch/1 -> u_I/1, Sum5/2  "u_I"
  I_Cntr_On/1 -> Switch/2
  Constant/1 -> Switch/3
  xC_Ref/1 -> Gain2/1
  Controller_Reset/1(I_Reset) -> I_reset/1, Discrete-Time Integrator/2
  Sum3/1 -> Divide/1
  Clock/1 -> Controller_Reset/1(Clock)
  Gain1/1 -> Sum1/2
  Gain2/1 -> Sum1/1
  Gain3/1 -> Pos_Error/1
  D_Den2/1 -> Vector Concatenate1/2
  D_Num2/1 -> Vector Concatenate/2
  Vector Concatenate/1 -> Discrete Transfer Fcn/2
  D_Num1/1 -> Vector Concatenate/1
  Vector Concatenate1/1 -> Discrete Transfer Fcn/3
  D_Den1/1 -> Vector Concatenate1/1
  Saturation2/1 -> u_FB/1
  Constant1/1 -> Switch1/3
  Saturation1/1 -> Switch1/1, Sum3/2
  Gain/1 -> Saturation2/1
  FB_Cntr_On/1 -> Switch1/2
  Switch1/1 -> Gain/1  "w_ref"
  Sum5/1 -> Saturation1/1, Sum3/1  "u_FB [-]"
  D_Cntr_On/1 -> Switch2/2
  Switch2/1 -> Sum5/3  "u_D"
  Constant2/1 -> Switch2/3
  Discrete Transfer Fcn/1 -> Switch2/1
  Sum1/1 -> Discrete Transfer Fcn/1, Product/2, Sum2/1, Gain3/1
  D_Den3/1 -> Vector Concatenate1/3

== system Function_Blocks/SCC_SinProfile ==
  Enable : Inport  OutDataTypeStr=boolean
  x0 : Inport  Port=2
  v0 : Inport  Port=3
  xC_SP : Inport  Port=4
  T : Inport  Port=5
  Clock : Inport  Port=6
  Constant : Constant  Value=0
  Constant1 : Constant  Value=pi
  Switch : Switch  Criteria=u2 > Threshold
  Switch1 : Switch  Criteria=u2 > Threshold
  WaveSignal : MATLAB Function  TreatAsAtomicUnit=on
  xC : Outport  VectorParamsAs1DForOutWhenUnconnected=off
  vC : Outport  Port=2  VectorParamsAs1DForOutWhenUnconnected=off
  wires:
  x0/1 -> WaveSignal/1(x0)
  T/1 -> WaveSignal/4(Ts)
  Clock/1 -> WaveSignal/6(t)
  xC_SP/1 -> WaveSignal/3(xC_SP)
  Constant1/1 -> WaveSignal/5(phi)
  v0/1 -> WaveSignal/2(v0)
  Switch/1 -> xC/1
  WaveSignal/1(x) -> Switch/1
  Constant/1 -> Switch1/3, Switch/3
  Switch1/1 -> vC/1
  Enable/1 -> Switch1/2, Switch/2
  WaveSignal/2(dx) -> Switch1/1

== system Function_Blocks/SCC_VFF  ==
  VFF_On : Inport  OutDataTypeStr=boolean
  kVFF : Inport  Port=2
  Aa : Inport  Port=3
  kq : Inport  Port=4
  v_ref_mms : Inport  Port=5
  Constant : Constant  Value=0
  Divide1 : Product  Inputs=*/
  Gain1 : Gain  Gain=1e-3
  Product : Product
  Product1 : Product
  Switch1 : Switch  Criteria=u2 > Threshold
  uFF : Outport  VectorParamsAs1DForOutWhenUnconnected=off
  wires:
  v_ref_mms/1 -> Gain1/1
  Gain1/1 -> Product1/2  "v_Set [m/s]"
  Product1/1 -> Divide1/1
  Switch1/1 -> uFF/1
  VFF_On/1 -> Switch1/2
  Constant/1 -> Switch1/3
  Divide1/1 -> Product/1
  Product/1 -> Switch1/1
  kVFF/1 -> Product/2
  kq/1 -> Divide1/2
  Aa/1 -> Product1/1

== system Function_Blocks/SCC_Vel_AD ==
  Enable : Inport  OutDataTypeStr=boolean
  2sDelay : Inport  Port=2
  HPF_Num1 : Inport  Port=3
  HPF_Num2 : Inport  Port=4
  HPF_Den1 : Inport  Port=5
  HPF_Den2 : Inport  Port=6
  xC_mm : Inport  Port=7
  Constant : Constant  Value=0
  Constant3 : Constant  Value=0
  Discrete Derivative2 : simulink/Discrete/Discrete Derivative  gainval=1.0  ICPrevScaledInput=0.0  OutMin=[]  OutMax=[]  OutDataType=fixdt(1, 16)  OutScaling=2^-10  DoSatur=off
  Gain : Gain  Gain=1e-3
  HP_Filter : DiscreteTransferFcn  NumeratorSource=Input port  Numerator=[3.786e-11 -3.786e-11]  DenominatorSource=Input port  Denominator=[1 -0.9954]  SampleTime=0.001  a0EqualsOne=on
      settings: InputPortMap=u0,p1,p3
  Low-Pass Filter (Discrete or Continuous)1 : eeGeneralControl/Low-Pass Filter (Discrete or Continuous)  K=1  T=0.1  B=0.175  A=-0.175  init_option=Inherited from block input  x0=0  Ts=0.001
  Saturation5 : Saturate  UpperLimit=3600  LowerLimit=-3600
  Switch1 : Switch  Criteria=u2 > Threshold  Threshold=2
  Switch2 : Switch  Criteria=u2 > Threshold
  Switch5 : Switch  Criteria=u2 > Threshold  Threshold=2
  Vector Concatenate : Concatenate
  Vector Concatenate1 : Concatenate
  uAD : Outport  VectorParamsAs1DForOutWhenUnconnected=off
  wires:
  xC_mm/1 -> Gain/1
  Constant/1 -> Switch2/3, Switch1/3
  Vector Concatenate/1 -> HP_Filter/2
  Vector Concatenate1/1 -> HP_Filter/3
  HPF_Num1/1 -> Vector Concatenate/1
  HPF_Num2/1 -> Vector Concatenate/2
  HPF_Den1/1 -> Vector Concatenate1/1
  HPF_Den2/1 -> Vector Concatenate1/2
  Switch2/1 -> Saturation5/1
  Switch1/1 -> Switch2/1
  Enable/1 -> Switch2/2
  Saturation5/1 -> uAD/1
  HP_Filter/1 -> Switch1/1
  Gain/1 -> Discrete Derivative2/1
  Discrete Derivative2/1 -> Low-Pass Filter (Discrete or Continuous)1/1
  Low-Pass Filter (Discrete or Continuous)1/1 -> Switch5/1
  Constant3/1 -> Switch5/3
  Switch5/1 -> HP_Filter/1
  2sDelay/1 -> Switch1/2, Switch5/2

== system Function_Blocks/S_shape_Profile ==
  Enable : Inport  OutDataTypeStr=boolean
  x0 : Inport  Port=2
  v0 : Inport  Port=3
  Position_SP : Inport  Port=4
  Velocity_SP : Inport  Port=5
  t0 : Inport  Port=6
  t_Hold_Position : Inport  Port=7
  CyclicTime : Inport  Port=8
  Constant : Constant  Value=0
  SP_Generator : MATLAB Function  TreatAsAtomicUnit=on
  Saturation : Saturate  UpperLimit=500  LowerLimit=0
  Saturation1 : Saturate  UpperLimit=150  LowerLimit=-150
  Saturation2 : Saturate  UpperLimit=150  LowerLimit=-150
  Saturation3 : Saturate  UpperLimit=500  LowerLimit=0
  Switch{,1..3} (4 alike) : Switch  Criteria=u2 > Threshold
  Position_Ref : Outport  VectorParamsAs1DForOutWhenUnconnected=off
  Velocity_Ref : Outport  Port=2  VectorParamsAs1DForOutWhenUnconnected=off
  Acceleration_Ref : Outport  Port=3  VectorParamsAs1DForOutWhenUnconnected=off
  Jerk_Ref : Outport  Port=4  VectorParamsAs1DForOutWhenUnconnected=off
  Motion_Cycle_Time : Outport  Port=5  VectorParamsAs1DForOutWhenUnconnected=off
  Error : Outport  Port=6  VectorParamsAs1DForOutWhenUnconnected=off
  wires:
  Saturation/1 -> SP_Generator/3(Desired_Position)
  Saturation1/1 -> SP_Generator/4(VelocitySP)
  t0/1 -> SP_Generator/5(t0)
  t_Hold_Position/1 -> SP_Generator/6(HoldPositionTime)
  Velocity_SP/1 -> Saturation1/1
  SP_Generator/5(InPositionTime) -> Motion_Cycle_Time/1
  CyclicTime/1 -> SP_Generator/7(t)
  SP_Generator/6(Error) -> Error/1
  Position_SP/1 -> Saturation/1
  Saturation2/1 -> Velocity_Ref/1
  Switch/1 -> Saturation2/1
  x0/1 -> Switch1/3, SP_Generator/1(s0)
  SP_Generator/1(PositionRef) -> Switch1/1
  Saturation3/1 -> Position_Ref/1
  v0/1 -> Switch/3, SP_Generator/2(v0)
  Enable/1 -> Switch1/2, Switch/2, Switch3/2, Switch2/2
  SP_Generator/2(VelocityRef) -> Switch/1
  Switch1/1 -> Saturation3/1
  SP_Generator/3(AccelerationRef) -> Switch2/1
  SP_Generator/4(JerkRef) -> Switch3/1
  Constant/1 -> Switch3/3, Switch2/3
  Switch2/1 -> Acceleration_Ref/1
  Switch3/1 -> Jerk_Ref/1

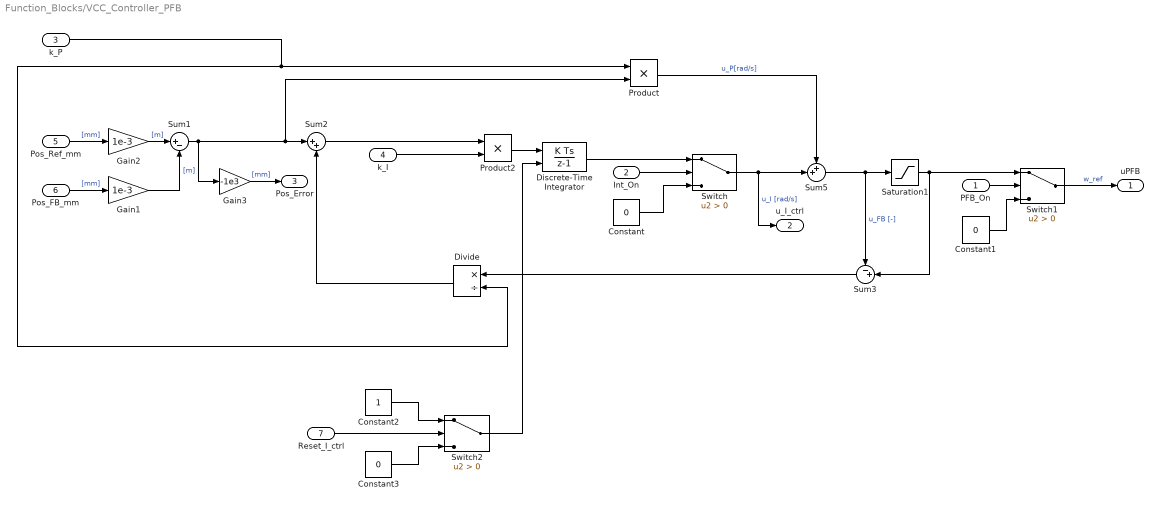
== system Function_Blocks/VCC_Controller_PFB ==
  PFB_On : Inport  OutDataTypeStr=boolean
  Int_On : Inport  Port=2  OutDataTypeStr=boolean
  k_P : Inport  Port=3
  k_I : Inport  Port=4
  Pos_Ref_mm : Inport  Port=5
  Pos_FB_mm : Inport  Port=6
  Reset_I_ctrl : Inport  Port=7  OutDataTypeStr=boolean
  Constant : Constant  Value=0
  Constant1 : Constant  Value=0
  Constant2 : Constant
  Constant3 : Constant  Value=0
  Discrete-Time Integrator : DiscreteIntegrator  ExternalReset=sampled level  SampleTime=0.001  ICPrevOutput=DiscIntNeverNeededParam  ICPrevScaledInput=DiscIntNeverNeededParam
  Divide : Product  Inputs=*/
  Gain1 : Gain  Gain=1e-3
  Gain2 : Gain  Gain=1e-3
  Gain3 : Gain  Gain=-1e3
  Product : Product
  Product2 : Product
  Saturation1 : Saturate  UpperLimit=1  LowerLimit=-1
  Sum1 : Sum  Inputs=|+-
  Sum2 : Sum  Inputs=|++
  Sum3 : Sum  Inputs=-+|
  Sum5 : Sum  Inputs=++|
  Switch : Switch  Criteria=u2 > Threshold
  Switch1 : Switch  Criteria=u2 > Threshold
  Switch2 : Switch  Criteria=u2 > Threshold
  uPFB : Outport  VectorParamsAs1DForOutWhenUnconnected=off
  u_I_ctrl : Outport  Port=2  VectorParamsAs1DForOutWhenUnconnected=off
  Pos_Error : Outport  Port=3  VectorParamsAs1DForOutWhenUnconnected=off
  wires:
  Pos_FB_mm/1 -> Gain1/1  "[mm]"
  Sum2/1 -> Product2/1
  Divide/1 -> Sum2/2
  k_P/1 -> Product/1, Divide/2
  k_I/1 -> Product2/2
  Sum1/1 -> Product/2, Sum2/1, Gain3/1
  Int_On/1 -> Switch/2
  Constant/1 -> Switch/3
  Pos_Ref_mm/1 -> Gain2/1  "[mm]"
  Sum5/1 -> Sum3/1, Saturation1/1  "u_FB [-]"
  Sum3/1 -> Divide/1
  Switch1/1 -> uPFB/1  "w_ref"
  Constant1/1 -> Switch1/3
  PFB_On/1 -> Switch1/2
  Saturation1/1 -> Switch1/1, Sum3/2
  Gain1/1 -> Sum1/2  "[m]"
  Gain2/1 -> Sum1/1  "[m]"
  Gain3/1 -> Pos_Error/1  "[mm]"
  Product/1 -> Sum5/1  "u_P[rad/s]"
  Switch/1 -> u_I_ctrl/1, Sum5/2  "u_I [rad/s]"
  Product2/1 -> Discrete-Time Integrator/1
  Reset_I_ctrl/1 -> Switch2/2
  Switch2/1 -> Discrete-Time Integrator/2
  Discrete-Time Integrator/1 -> Switch/1
  Constant2/1 -> Switch2/1
  Constant3/1 -> Switch2/3

== system Function_Blocks/VCC_Pos_Step ==
  Enable : Inport  OutDataTypeStr=boolean
  x0 : Inport  Port=2
  xSP : Inport  Port=3
  t0 : Inport  Port=4
  tHold : Inport  Port=5
  Clock : Inport  Port=6
  Constant : Constant  Value=0
  StepFunction : MATLAB Function  TreatAsAtomicUnit=on
  Switch : Switch  Criteria=u2 > Threshold
  xC_ref : Outport  VectorParamsAs1DForOutWhenUnconnected=off
  wires:
  Clock/1 -> StepFunction/5(t)
  x0/1 -> StepFunction/1(x0)
  StepFunction/1(y) -> Switch/1
  Switch/1 -> xC_ref/1
  Constant/1 -> Switch/3
  Enable/1 -> Switch/2
  xSP/1 -> StepFunction/2(x_SP)
  t0/1 -> StepFunction/3(t0)
  tHold/1 -> StepFunction/4(t1)

== system Function_Blocks/VCC_VFF ==
  Enable : Inport  OutDataTypeStr=boolean
  v_ref : Inport  Port=2
  Qmax : Inport  Port=3
  Annnulus_Area : Constant  Value=2356.2
  Bore_Area : Constant  Value=3318.3
  Constant : Constant  Value=0
  Divide2 : Product  Inputs=*/
  Gain1 : Gain  Gain=60000
  Gain3 : Gain  Gain=1e-9
  Product1 : Product
  Product3 : Product
  Switch1 : Switch  Criteria=u2 > Threshold
  Switch2 : Switch
  u_FF [-] : Outport  VectorParamsAs1DForOutWhenUnconnected=off
  wires:
  Annnulus_Area/1 -> Product3/2  "[mm^2]"
  Switch2/1 -> Gain3/1  "Q_ref [mm^3/s]"
  Product1/1 -> Switch2/1
  v_ref/1 -> Product3/1, Product1/2, Switch2/2
  Qmax/1 -> Divide2/2
  Bore_Area/1 -> Product1/1  "[mm^2]"
  Gain1/1 -> Divide2/1  "Q_ref [L/min]"
  Gain3/1 -> Gain1/1  "Q_ref [m^3/s]"
  Product3/1 -> Switch2/3
  Constant/1 -> Switch1/3
  Divide2/1 -> Switch1/1
  Switch1/1 -> u_FF [-]/1
  Enable/1 -> Switch1/2

== system Function_Blocks/VCC_VFF1 ==
  Enable : Inport  OutDataTypeStr=boolean
  v_ref : Inport  Port=2
  Qmax : Inport  Port=3
  Qmax1 : Inport  Port=4
  Annnulus_Area : Constant  Value=2356.2
  Bore_Area : Constant  Value=3318.3
  Constant : Constant  Value=0
  Divide2 : Product  Inputs=*/
  Gain1 : Gain  Gain=60000
  Gain3 : Gain  Gain=1e-9
  Product1 : Product
  Product3 : Product
  Switch1 : Switch  Criteria=u2 > Threshold
  Switch2 : Switch
  u_FF [-] : Outport  VectorParamsAs1DForOutWhenUnconnected=off
  wires:
  Annnulus_Area/1 -> Product3/2  "[mm^2]"
  Switch2/1 -> Gain3/1  "Q_ref [mm^3/s]"
  Product1/1 -> Switch2/1
  v_ref/1 -> Product3/1, Product1/2, Switch2/2
  Qmax/1 -> Divide2/2
  Bore_Area/1 -> Product1/1  "[mm^2]"
  Gain1/1 -> Divide2/1  "Q_ref [L/min]"
  Gain3/1 -> Gain1/1  "Q_ref [m^3/s]"
  Product3/1 -> Switch2/3
  Constant/1 -> Switch1/3
  Divide2/1 -> Switch1/1
  Switch1/1 -> u_FF [-]/1
  Enable/1 -> Switch1/2

== system Function_Blocks/Cylinder Controller/I_Reset1 ==
  Position_Error : Inport
  Vel_SP : Inport  Port=2
  Abs : Abs
  Abs1 : Abs
  Constant1 : Constant  Value=0
  Constant2 : Constant
  Constant5 : Constant
  Constant6 : Constant  Value=0
  Product : Product
  Switch1 : Switch  Criteria=u2 > Threshold  Threshold=Error_Limit
  Switch2 : Switch  Criteria=u2 > Threshold
  Reset : Outport  VectorParamsAs1DForOutWhenUnconnected=off
  wires:
  Position_Error/1 -> Abs/1
  Constant6/1 -> Switch1/1
  Constant5/1 -> Switch1/3
  Abs/1 -> Switch1/2
  Abs1/1 -> Switch2/2
  Constant1/1 -> Switch2/1
  Constant2/1 -> Switch2/3
  Switch1/1 -> Product/1
  Switch2/1 -> Product/2
  Product/1 -> Reset/1
  Vel_SP/1 -> Abs1/1
